simulink model "simscape"  (R2020b)
settings: Solver=VariableStepAuto  StartTime=0.0  StopTime=10.0  RelTol=1e-3
settings Model: Creator=SOREN  LastModifiedBy=SOREN

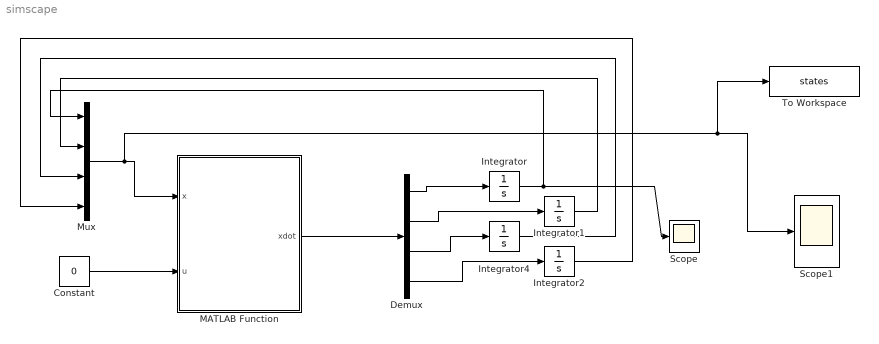
== system simscape ==
  Constant : Constant  Value=0
  Demux : Demux
  Integrator : Integrator  InitialCondition=1
  Integrator1 : Integrator
  Integrator2 : Integrator
  Integrator4 : Integrator
  MATLAB Function : MATLAB Function  TreatAsAtomicUnit=on
  Mux : Mux
  Scope : Scope
  Scope1 : Scope
  To Workspace : ToWorkspace  VariableName=states  SampleTime=-1
  wires:
  Constant/1 -> MATLAB Function/2(u)
  MATLAB Function/1(xdot) -> Demux/1
  Demux/1 -> Integrator/1
  Demux/3 -> Integrator4/1
  Demux/2 -> Integrator1/1
  Integrator1/1 -> Mux/2
  Integrator/1 -> Scope/1, Mux/1
  Integrator4/1 -> Mux/3
  Integrator2/1 -> Mux/4
  Mux/1 -> To Workspace/1, Scope1/1, MATLAB Function/1(x)
  Demux/4 -> Integrator2/1

== matlab function simscape/MATLAB Function ==
  data: x input; u input; xdot output
function xdot = integral_controller(x,u)
A = [-110 -2400 -1.04e5 0;
     1 0 0 0;
     0 1 0 0;
     0 0 1 0];
 
B = [1; 0;0; 0];
C = [0 0 0 2000000]; % Output matrix to observe all states
D = 0;

xdot = A*x + B*u ; %without disturbance
